simulink model "x12_agv"  (R2025a)
settings: Solver=VariableStepAuto  StartTime=0.0  StopTime=30  RelTol=1e-3
undefined symbols (not defined in the file): Ad, Bd, d_sel, K, kc_pos, kc_vel, p, ref_1, ref_10, ref_11, ref_12, ref_2, ref_3, ref_4, ref_5, ref_6, ref_7, ref_8, ref_9, Ts, x0, x0_1, x0_10, x0_11, x0_12, x0_2, x0_3, x0_4, x0_5, x0_6, x0_7, x0_8, x0_9
(part 1 of 2)
settings Model: Creator=pc  LastModifiedBy=pc

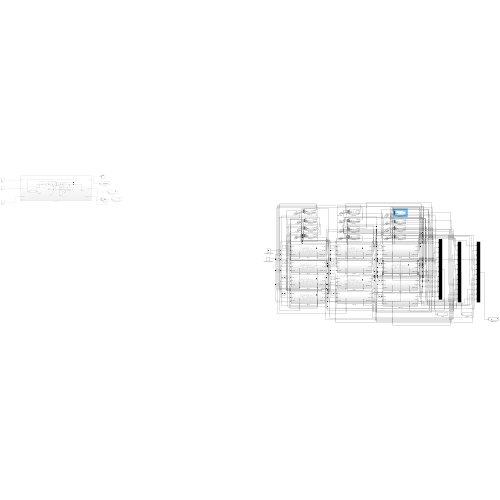
[thumbnail: Simulink's stored preview of the top-level diagram]
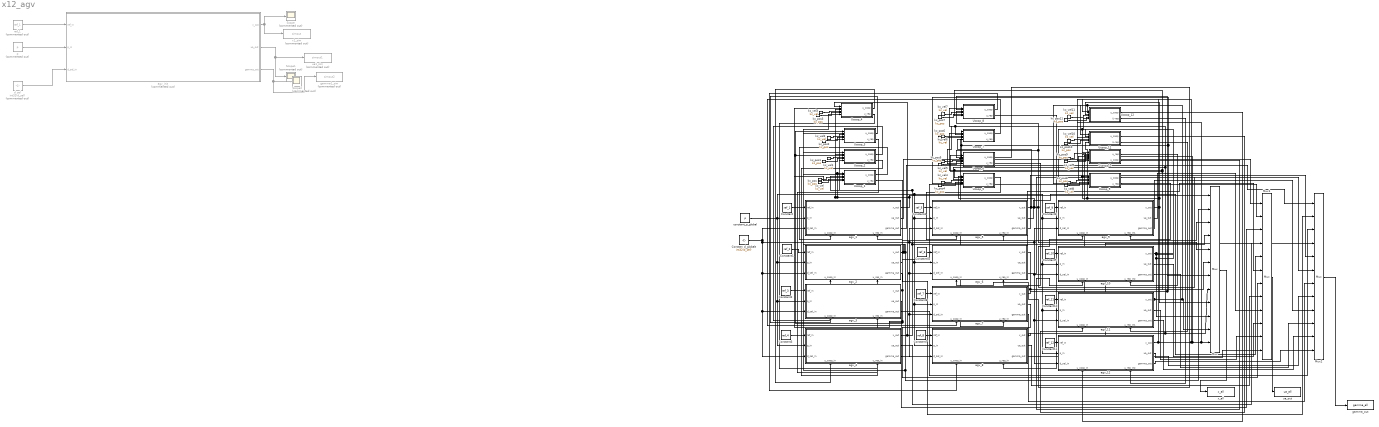
== system x12_agv ==
  Constan_d_globalt : Constant  Value=int32(d_sel)
  Constant : Constant  Value=ref_1
  Constant1 : Constant  Value=ref_2
  Constant10 : Constant  Value=ref_11
  Constant11 : Constant  Value=ref_12
  Constant2 : Constant  Value=ref_3
  Constant3 : Constant  Value=ref_4
  Constant4 : Constant  Value=ref_5
  Constant5 : Constant  Value=ref_6
  Constant6 : Constant  Value=ref_7
  Constant7 : Constant  Value=ref_8
  Constant8 : Constant  Value=ref_9
  Constant9 : Constant  Value=ref_10
  Mux : Mux  Inputs=12
  Mux1 : Mux  Inputs=12
  Mux2 : Mux  Inputs=12
  Scope : Scope  Commented=on
      settings: ActiveDisplayYMinimum=-8.609830640918906  ActiveDisplayYMaximum=10.643757487994291
  Scope1 : Scope  Commented=on
      settings: ActiveDisplayYMinimum=-1.4791031893143503  ActiveDisplayYMaximum=0.83872011794707424
  Scope2 : Scope  Commented=on
      settings: ActiveDisplayYMinimum=-0.20234469315895376  ActiveDisplayYMaximum=1.2446865568410463  DataLoggingVariableName=ScopeData2
  Ucoop_1 : Subsystem
  Ucoop_10 : Subsystem
  Ucoop_11 : Subsystem
  Ucoop_12 : Subsystem
  Ucoop_2 : Subsystem
  Ucoop_3 : Subsystem
  Ucoop_4 : Subsystem
  Ucoop_5 : Subsystem
  Ucoop_6 : Subsystem
  Ucoop_7 : Subsystem
  Ucoop_8 : Subsystem
  Ucoop_9 : Subsystem
  agv_1 : Subsystem
      settings: PortSchema="{\"entries\":[{\"content\":{\"sides\":[{\"content\":{\"connectorIds\":[\"In1\",\"In2\",\"In3\"]},\"type\":\"ConnectorPlacement.EquallySpacedRectSide\",\"uuid\":\"f08cf805-8739-441b-9df1-afc331da9c66\"},{\"content\":{\"connectorIds\":[\"Out1\",\"Out2\",\"Out3\"],\"side\":\"RIGHT\"},\"type\":\"ConnectorPlacement.EquallySpacedRectSide\",\"uuid\":\"8dfbec97-d8e8-49f2-8859-a95f098f15d4\"},{\"content\":{\"side\":\"TOP\"},\"type\":\"ConnectorPlacement.EquallySpacedRectSide\",\"uuid\":\"a9c3710a-c537-4e60-ba39-fa8e56fd912a\"},{\"content\":{\"connectorIds\":[\"In4\",\"In5\"],\"side\":\"BOTTOM\"},\"type\":\"ConnectorPlacement.EquallySpacedRectSide\",\"uuid\":\"8d7992a2-b8d6-4781-b503-987242c7d025\"}]},\"type\":\"ConnectorPlacement.EquallySpacedConnector\",\"uuid\":\"d7bc182e-c1cf-4fe9-ae71-f4bbcf9bd096\"}],\"packageUris\":[\"http://schema.mathworks.com/mf0/Connector/R2020b\"],\"version\":\"1.0\"}"
  agv_10 : Subsystem
      settings: PortSchema="{\"entries\":[{\"content\":{\"sides\":[{\"content\":{\"connectorIds\":[\"In1\",\"In2\",\"In3\"]},\"type\":\"ConnectorPlacement.EquallySpacedRectSide\",\"uuid\":\"f08cf805-8739-441b-9df1-afc331da9c66\"},{\"content\":{\"connectorIds\":[\"Out1\",\"Out2\",\"Out3\"],\"side\":\"RIGHT\"},\"type\":\"ConnectorPlacement.EquallySpacedRectSide\",\"uuid\":\"8dfbec97-d8e8-49f2-8859-a95f098f15d4\"},{\"content\":{\"side\":\"TOP\"},\"type\":\"ConnectorPlacement.EquallySpacedRectSide\",\"uuid\":\"a9c3710a-c537-4e60-ba39-fa8e56fd912a\"},{\"content\":{\"connectorIds\":[\"In4\",\"In5\"],\"side\":\"BOTTOM\"},\"type\":\"ConnectorPlacement.EquallySpacedRectSide\",\"uuid\":\"65549514-36e3-47a4-b89a-5d3e141dfba9\"}]},\"type\":\"ConnectorPlacement.EquallySpacedConnector\",\"uuid\":\"d7bc182e-c1cf-4fe9-ae71-f4bbcf9bd096\"}],\"packageUris\":[\"http://schema.mathworks.com/mf0/Connector/R2020b\"],\"version\":\"1.0\"}"
  agv_11 : Subsystem
      settings: PortSchema="{\"entries\":[{\"content\":{\"sides\":[{\"content\":{\"connectorIds\":[\"In1\",\"In2\",\"In3\"]},\"type\":\"ConnectorPlacement.EquallySpacedRectSide\",\"uuid\":\"f08cf805-8739-441b-9df1-afc331da9c66\"},{\"content\":{\"connectorIds\":[\"Out1\",\"Out2\",\"Out3\"],\"side\":\"RIGHT\"},\"type\":\"ConnectorPlacement.EquallySpacedRectSide\",\"uuid\":\"8dfbec97-d8e8-49f2-8859-a95f098f15d4\"},{\"content\":{\"side\":\"TOP\"},\"type\":\"ConnectorPlacement.EquallySpacedRectSide\",\"uuid\":\"a9c3710a-c537-4e60-ba39-fa8e56fd912a\"},{\"content\":{\"connectorIds\":[\"In4\",\"In5\"],\"side\":\"BOTTOM\"},\"type\":\"ConnectorPlacement.EquallySpacedRectSide\",\"uuid\":\"8d7992a2-b8d6-4781-b503-987242c7d025\"}]},\"type\":\"ConnectorPlacement.EquallySpacedConnector\",\"uuid\":\"d7bc182e-c1cf-4fe9-ae71-f4bbcf9bd096\"}],\"packageUris\":[\"http://schema.mathworks.com/mf0/Connector/R2020b\"],\"version\":\"1.0\"}"
  agv_12 : Subsystem
      settings: PortSchema="{\"entries\":[{\"content\":{\"sides\":[{\"content\":{\"connectorIds\":[\"In1\",\"In2\",\"In3\"]},\"type\":\"ConnectorPlacement.EquallySpacedRectSide\",\"uuid\":\"f08cf805-8739-441b-9df1-afc331da9c66\"},{\"content\":{\"connectorIds\":[\"Out1\",\"Out2\",\"Out3\"],\"side\":\"RIGHT\"},\"type\":\"ConnectorPlacement.EquallySpacedRectSide\",\"uuid\":\"8dfbec97-d8e8-49f2-8859-a95f098f15d4\"},{\"content\":{\"side\":\"TOP\"},\"type\":\"ConnectorPlacement.EquallySpacedRectSide\",\"uuid\":\"a9c3710a-c537-4e60-ba39-fa8e56fd912a\"},{\"content\":{\"connectorIds\":[\"In4\",\"In5\"],\"side\":\"BOTTOM\"},\"type\":\"ConnectorPlacement.EquallySpacedRectSide\",\"uuid\":\"8d7992a2-b8d6-4781-b503-987242c7d025\"}]},\"type\":\"ConnectorPlacement.EquallySpacedConnector\",\"uuid\":\"d7bc182e-c1cf-4fe9-ae71-f4bbcf9bd096\"}],\"packageUris\":[\"http://schema.mathworks.com/mf0/Connector/R2020b\"],\"version\":\"1.0\"}"
  agv_2 : Subsystem
      settings: PortSchema="{\"entries\":[{\"content\":{\"sides\":[{\"content\":{\"connectorIds\":[\"In1\",\"In2\",\"In3\"]},\"type\":\"ConnectorPlacement.EquallySpacedRectSide\",\"uuid\":\"f08cf805-8739-441b-9df1-afc331da9c66\"},{\"content\":{\"connectorIds\":[\"Out1\",\"Out2\",\"Out3\"],\"side\":\"RIGHT\"},\"type\":\"ConnectorPlacement.EquallySpacedRectSide\",\"uuid\":\"8dfbec97-d8e8-49f2-8859-a95f098f15d4\"},{\"content\":{\"side\":\"TOP\"},\"type\":\"ConnectorPlacement.EquallySpacedRectSide\",\"uuid\":\"a9c3710a-c537-4e60-ba39-fa8e56fd912a\"},{\"content\":{\"connectorIds\":[\"In4\",\"In5\"],\"side\":\"BOTTOM\"},\"type\":\"ConnectorPlacement.EquallySpacedRectSide\",\"uuid\":\"65549514-36e3-47a4-b89a-5d3e141dfba9\"}]},\"type\":\"ConnectorPlacement.EquallySpacedConnector\",\"uuid\":\"d7bc182e-c1cf-4fe9-ae71-f4bbcf9bd096\"}],\"packageUris\":[\"http://schema.mathworks.com/mf0/Connector/R2020b\"],\"version\":\"1.0\"}"
  agv_3 : Subsystem
      settings: PortSchema="{\"entries\":[{\"content\":{\"sides\":[{\"content\":{\"connectorIds\":[\"In1\",\"In2\",\"In3\"]},\"type\":\"ConnectorPlacement.EquallySpacedRectSide\",\"uuid\":\"f08cf805-8739-441b-9df1-afc331da9c66\"},{\"content\":{\"connectorIds\":[\"Out1\",\"Out2\",\"Out3\"],\"side\":\"RIGHT\"},\"type\":\"ConnectorPlacement.EquallySpacedRectSide\",\"uuid\":\"8dfbec97-d8e8-49f2-8859-a95f098f15d4\"},{\"content\":{\"side\":\"TOP\"},\"type\":\"ConnectorPlacement.EquallySpacedRectSide\",\"uuid\":\"a9c3710a-c537-4e60-ba39-fa8e56fd912a\"},{\"content\":{\"connectorIds\":[\"In4\",\"In5\"],\"side\":\"BOTTOM\"},\"type\":\"ConnectorPlacement.EquallySpacedRectSide\",\"uuid\":\"8d7992a2-b8d6-4781-b503-987242c7d025\"}]},\"type\":\"ConnectorPlacement.EquallySpacedConnector\",\"uuid\":\"d7bc182e-c1cf-4fe9-ae71-f4bbcf9bd096\"}],\"packageUris\":[\"http://schema.mathworks.com/mf0/Connector/R2020b\"],\"version\":\"1.0\"}"
  agv_4 : Subsystem
      settings: PortSchema="{\"entries\":[{\"content\":{\"sides\":[{\"content\":{\"connectorIds\":[\"In1\",\"In2\",\"In3\"]},\"type\":\"ConnectorPlacement.EquallySpacedRectSide\",\"uuid\":\"f08cf805-8739-441b-9df1-afc331da9c66\"},{\"content\":{\"connectorIds\":[\"Out1\",\"Out2\",\"Out3\"],\"side\":\"RIGHT\"},\"type\":\"ConnectorPlacement.EquallySpacedRectSide\",\"uuid\":\"8dfbec97-d8e8-49f2-8859-a95f098f15d4\"},{\"content\":{\"side\":\"TOP\"},\"type\":\"ConnectorPlacement.EquallySpacedRectSide\",\"uuid\":\"a9c3710a-c537-4e60-ba39-fa8e56fd912a\"},{\"content\":{\"connectorIds\":[\"In4\",\"In5\"],\"side\":\"BOTTOM\"},\"type\":\"ConnectorPlacement.EquallySpacedRectSide\",\"uuid\":\"8d7992a2-b8d6-4781-b503-987242c7d025\"}]},\"type\":\"ConnectorPlacement.EquallySpacedConnector\",\"uuid\":\"d7bc182e-c1cf-4fe9-ae71-f4bbcf9bd096\"}],\"packageUris\":[\"http://schema.mathworks.com/mf0/Connector/R2020b\"],\"version\":\"1.0\"}"
  agv_5 : Subsystem
      settings: PortSchema="{\"entries\":[{\"content\":{\"sides\":[{\"content\":{\"connectorIds\":[\"In1\",\"In2\",\"In3\"]},\"type\":\"ConnectorPlacement.EquallySpacedRectSide\",\"uuid\":\"f08cf805-8739-441b-9df1-afc331da9c66\"},{\"content\":{\"connectorIds\":[\"Out1\",\"Out2\",\"Out3\"],\"side\":\"RIGHT\"},\"type\":\"ConnectorPlacement.EquallySpacedRectSide\",\"uuid\":\"8dfbec97-d8e8-49f2-8859-a95f098f15d4\"},{\"content\":{\"side\":\"TOP\"},\"type\":\"ConnectorPlacement.EquallySpacedRectSide\",\"uuid\":\"a9c3710a-c537-4e60-ba39-fa8e56fd912a\"},{\"content\":{\"connectorIds\":[\"In4\",\"In5\"],\"side\":\"BOTTOM\"},\"type\":\"ConnectorPlacement.EquallySpacedRectSide\",\"uuid\":\"8d7992a2-b8d6-4781-b503-987242c7d025\"}]},\"type\":\"ConnectorPlacement.EquallySpacedConnector\",\"uuid\":\"d7bc182e-c1cf-4fe9-ae71-f4bbcf9bd096\"}],\"packageUris\":[\"http://schema.mathworks.com/mf0/Connector/R2020b\"],\"version\":\"1.0\"}"
  agv_6 : Subsystem
      settings: PortSchema="{\"entries\":[{\"content\":{\"sides\":[{\"content\":{\"connectorIds\":[\"In1\",\"In2\",\"In3\"]},\"type\":\"ConnectorPlacement.EquallySpacedRectSide\",\"uuid\":\"f08cf805-8739-441b-9df1-afc331da9c66\"},{\"content\":{\"connectorIds\":[\"Out1\",\"Out2\",\"Out3\"],\"side\":\"RIGHT\"},\"type\":\"ConnectorPlacement.EquallySpacedRectSide\",\"uuid\":\"8dfbec97-d8e8-49f2-8859-a95f098f15d4\"},{\"content\":{\"side\":\"TOP\"},\"type\":\"ConnectorPlacement.EquallySpacedRectSide\",\"uuid\":\"a9c3710a-c537-4e60-ba39-fa8e56fd912a\"},{\"content\":{\"connectorIds\":[\"In4\",\"In5\"],\"side\":\"BOTTOM\"},\"type\":\"ConnectorPlacement.EquallySpacedRectSide\",\"uuid\":\"65549514-36e3-47a4-b89a-5d3e141dfba9\"}]},\"type\":\"ConnectorPlacement.EquallySpacedConnector\",\"uuid\":\"d7bc182e-c1cf-4fe9-ae71-f4bbcf9bd096\"}],\"packageUris\":[\"http://schema.mathworks.com/mf0/Connector/R2020b\"],\"version\":\"1.0\"}"
  agv_7 : Subsystem
      settings: PortSchema="{\"entries\":[{\"content\":{\"sides\":[{\"content\":{\"connectorIds\":[\"In1\",\"In2\",\"In3\"]},\"type\":\"ConnectorPlacement.EquallySpacedRectSide\",\"uuid\":\"f08cf805-8739-441b-9df1-afc331da9c66\"},{\"content\":{\"connectorIds\":[\"Out1\",\"Out2\",\"Out3\"],\"side\":\"RIGHT\"},\"type\":\"ConnectorPlacement.EquallySpacedRectSide\",\"uuid\":\"8dfbec97-d8e8-49f2-8859-a95f098f15d4\"},{\"content\":{\"side\":\"TOP\"},\"type\":\"ConnectorPlacement.EquallySpacedRectSide\",\"uuid\":\"a9c3710a-c537-4e60-ba39-fa8e56fd912a\"},{\"content\":{\"connectorIds\":[\"In4\",\"In5\"],\"side\":\"BOTTOM\"},\"type\":\"ConnectorPlacement.EquallySpacedRectSide\",\"uuid\":\"8d7992a2-b8d6-4781-b503-987242c7d025\"}]},\"type\":\"ConnectorPlacement.EquallySpacedConnector\",\"uuid\":\"d7bc182e-c1cf-4fe9-ae71-f4bbcf9bd096\"}],\"packageUris\":[\"http://schema.mathworks.com/mf0/Connector/R2020b\"],\"version\":\"1.0\"}"
  agv_8 : Subsystem
      settings: PortSchema="{\"entries\":[{\"content\":{\"sides\":[{\"content\":{\"connectorIds\":[\"In1\",\"In2\",\"In3\"]},\"type\":\"ConnectorPlacement.EquallySpacedRectSide\",\"uuid\":\"f08cf805-8739-441b-9df1-afc331da9c66\"},{\"content\":{\"connectorIds\":[\"Out1\",\"Out2\",\"Out3\"],\"side\":\"RIGHT\"},\"type\":\"ConnectorPlacement.EquallySpacedRectSide\",\"uuid\":\"8dfbec97-d8e8-49f2-8859-a95f098f15d4\"},{\"content\":{\"side\":\"TOP\"},\"type\":\"ConnectorPlacement.EquallySpacedRectSide\",\"uuid\":\"a9c3710a-c537-4e60-ba39-fa8e56fd912a\"},{\"content\":{\"connectorIds\":[\"In4\",\"In5\"],\"side\":\"BOTTOM\"},\"type\":\"ConnectorPlacement.EquallySpacedRectSide\",\"uuid\":\"8d7992a2-b8d6-4781-b503-987242c7d025\"}]},\"type\":\"ConnectorPlacement.EquallySpacedConnector\",\"uuid\":\"d7bc182e-c1cf-4fe9-ae71-f4bbcf9bd096\"}],\"packageUris\":[\"http://schema.mathworks.com/mf0/Connector/R2020b\"],\"version\":\"1.0\"}"
  agv_9 : Subsystem
      settings: PortSchema="{\"entries\":[{\"content\":{\"sides\":[{\"content\":{\"connectorIds\":[\"In1\",\"In2\",\"In3\"]},\"type\":\"ConnectorPlacement.EquallySpacedRectSide\",\"uuid\":\"f08cf805-8739-441b-9df1-afc331da9c66\"},{\"content\":{\"connectorIds\":[\"Out1\",\"Out2\",\"Out3\"],\"side\":\"RIGHT\"},\"type\":\"ConnectorPlacement.EquallySpacedRectSide\",\"uuid\":\"8dfbec97-d8e8-49f2-8859-a95f098f15d4\"},{\"content\":{\"side\":\"TOP\"},\"type\":\"ConnectorPlacement.EquallySpacedRectSide\",\"uuid\":\"a9c3710a-c537-4e60-ba39-fa8e56fd912a\"},{\"content\":{\"connectorIds\":[\"In4\",\"In5\"],\"side\":\"BOTTOM\"},\"type\":\"ConnectorPlacement.EquallySpacedRectSide\",\"uuid\":\"8d7992a2-b8d6-4781-b503-987242c7d025\"}]},\"type\":\"ConnectorPlacement.EquallySpacedConnector\",\"uuid\":\"d7bc182e-c1cf-4fe9-ae71-f4bbcf9bd096\"}],\"packageUris\":[\"http://schema.mathworks.com/mf0/Connector/R2020b\"],\"version\":\"1.0\"}"
  agv_init : Subsystem  Commented=on
  constant_p_global : Constant  Value=p
  d_sel : Constant  Commented=on  Value=int32(d_sel)
  gamma1_sim : ToWorkspace  Commented=on  VariableName=simout2  SaveFormat=Timeseries  SampleTime=-1
  gamma_out : ToWorkspace  VariableName=gamma_all  SaveFormat=Timeseries  SampleTime=-1
  kc_pos{,1..11} (12 alike) : Constant  Value=kc_pos
  kc_vel{,1..11} (12 alike) : Constant  Value=kc_vel
  p : Constant  Commented=on  Value=p
  ref_1 : Constant  Commented=on  Value=ref_1
  ua1_sim : ToWorkspace  Commented=on  VariableName=simout1  SaveFormat=Timeseries  SampleTime=-1
  ua_out : ToWorkspace  VariableName=ua_all  SaveFormat=Timeseries  SampleTime=-1
  x1_sim : ToWorkspace  Commented=on  VariableName=simout  SaveFormat=Timeseries  SampleTime=-1
  x_all : ToWorkspace  VariableName=x_all  SaveFormat=Timeseries  SampleTime=-1
  wires:
  agv_init/1(x_out) -> Scope/1, x1_sim/1
  agv_init/2(ua_out) -> Scope1/1, ua1_sim/1
  agv_init/3(gamma_out) -> gamma1_sim/1, Scope2/1
  ref_1/1 -> agv_init/1(ref_in)
  p/1 -> agv_init/2(p_in)
  d_sel/1 -> agv_init/3(d_sel_in)
  constant_p_global/1 -> agv_9/2(p_in), agv_10/2(p_in), agv_12/2(p_in), agv_11/2(p_in), agv_5/2(p_in), agv_6/2(p_in), agv_8/2(p_in), agv_7/2(p_in), agv_1/2(p_in), agv_2/2(p_in), agv_4/2(p_in), agv_3/2(p_in)
  Constan_d_globalt/1 -> agv_5/3(d_sel_in), agv_9/3(d_sel_in), agv_10/3(d_sel_in), agv_12/3(d_sel_in), agv_11/3(d_sel_in), agv_6/3(d_sel_in), agv_8/3(d_sel_in), agv_7/3(d_sel_in), agv_2/3(d_sel_in), agv_4/3(d_sel_in), agv_3/3(d_sel_in), agv_1/3(d_sel_in)
  Constant/1 -> agv_1/1(ref_in)
  Constant1/1 -> agv_2/1(ref_in)
  Constant2/1 -> agv_3/1(ref_in)
  Constant3/1 -> agv_4/1(ref_in)
  Constant4/1 -> agv_5/1(ref_in)
  Constant5/1 -> agv_6/1(ref_in)
  Constant6/1 -> agv_7/1(ref_in)
  Constant7/1 -> agv_8/1(ref_in)
  Constant8/1 -> agv_9/1(ref_in)
  Constant9/1 -> agv_10/1(ref_in)
  Constant10/1 -> agv_11/1(ref_in)
  Constant11/1 -> agv_12/1(ref_in)
  agv_1/1(x_out) -> Ucoop_3/6(xj3), Ucoop_4/3(xj2), Ucoop_2/2(xj1), Ucoop_1/1(xi), Mux/1
  agv_2/1(x_out) -> Ucoop_4/6(xj3), Mux/2, Ucoop_3/2(xj1), Ucoop_1/2(xj1), Ucoop_2/1(xi)
  agv_3/1(x_out) -> Ucoop_1/6(xj3), Ucoop_4/2(xj1), Ucoop_3/1(xi), Ucoop_2/3(xj2), Mux/3
  agv_4/1(x_out) -> Ucoop_2/6(xj3), Ucoop_3/3(xj2), Mux/4, Ucoop_4/1(xi), Ucoop_1/3(xj2)
  agv_5/1(x_out) -> Ucoop_7/6(xj3), Ucoop_8/3(xj2), Ucoop_6/2(xj1), Mux/5, Ucoop_5/1(xi)
  agv_6/1(x_out) -> Ucoop_8/6(xj3), Ucoop_5/2(xj1), Ucoop_7/2(xj1), Ucoop_6/1(xi), Mux/6
  agv_7/1(x_out) -> Ucoop_5/6(xj3), Ucoop_7/1(xi), Ucoop_6/3(xj2), Ucoop_8/2(xj1), Mux/7
  agv_8/1(x_out) -> Ucoop_8/1(xi), Ucoop_5/3(xj2), Mux/8, Ucoop_6/6(xj3), Ucoop_7/3(xj2)
  agv_9/1(x_out) -> Ucoop_11/6(xj3), Ucoop_10/2(xj1), Ucoop_9/1(xi), Ucoop_12/3(xj2), Mux/9
  agv_10/1(x_out) -> Ucoop_12/6(xj3), Ucoop_11/2(xj1), Mux/10, Ucoop_10/1(xi), Ucoop_9/2(xj1)
  agv_11/1(x_out) -> Ucoop_9/6(xj3), Mux/11, Ucoop_12/2(xj1), Ucoop_11/1(xi), Ucoop_10/3(xj2)
  agv_12/1(x_out) -> Ucoop_10/6(xj3), Ucoop_12/1(xi), Ucoop_9/3(xj2), Ucoop_11/3(xj2), Mux/12
  Mux/1 -> x_all/1
  agv_1/2(ua_out) -> Mux1/1
  agv_2/2(ua_out) -> Mux1/2
  agv_3/2(ua_out) -> Mux1/3
  agv_4/2(ua_out) -> Mux1/4
  agv_5/2(ua_out) -> Mux1/5
  agv_6/2(ua_out) -> Mux1/6
  agv_7/2(ua_out) -> Mux1/7
  agv_8/2(ua_out) -> Mux1/8
  agv_9/2(ua_out) -> Mux1/9
  agv_10/2(ua_out) -> Mux1/10
  agv_11/2(ua_out) -> Mux1/11
  agv_12/2(ua_out) -> Mux1/12
  Mux1/1 -> ua_out/1
  agv_1/3(gamma_out) -> Mux2/1
  agv_2/3(gamma_out) -> Mux2/2
  agv_3/3(gamma_out) -> Mux2/3
  agv_4/3(gamma_out) -> Mux2/4
  agv_5/3(gamma_out) -> Mux2/5
  agv_6/3(gamma_out) -> Mux2/6
  agv_7/3(gamma_out) -> Mux2/7
  agv_8/3(gamma_out) -> Mux2/8
  agv_9/3(gamma_out) -> Mux2/9
  agv_10/3(gamma_out) -> Mux2/10
  agv_11/3(gamma_out) -> Mux2/11
  agv_12/3(gamma_out) -> Mux2/12
  Mux2/1 -> gamma_out/1
  Ucoop_1/1(u_coop) -> agv_1/4(u_coop_in)
  kc_pos/1 -> Ucoop_1/5(kc_pos)
  kc_vel/1 -> Ucoop_1/4(kc_vel)
  kc_pos1/1 -> Ucoop_2/5(kc_pos)
  kc_vel1/1 -> Ucoop_2/4(kc_vel)
  kc_vel2/1 -> Ucoop_3/4(kc_vel)
  kc_pos2/1 -> Ucoop_3/5(kc_pos)
  Ucoop_2/1(u_coop) -> agv_2/4(u_coop_in)
  Ucoop_3/1(u_coop) -> agv_3/4(u_coop_in)
  kc_vel3/1 -> Ucoop_4/4(kc_vel)
  kc_pos3/1 -> Ucoop_4/5(kc_pos)
  Ucoop_4/1(u_coop) -> agv_4/4(u_coop_in)
  kc_vel4/1 -> Ucoop_5/4(kc_vel)
  kc_pos4/1 -> Ucoop_5/5(kc_pos)
  kc_vel5/1 -> Ucoop_6/4(kc_vel)
  kc_pos5/1 -> Ucoop_6/5(kc_pos)
  kc_vel6/1 -> Ucoop_7/4(kc_vel)
  kc_pos6/1 -> Ucoop_7/5(kc_pos)
  kc_vel7/1 -> Ucoop_8/4(kc_vel)
  kc_pos7/1 -> Ucoop_8/5(kc_pos)
  kc_vel8/1 -> Ucoop_9/4(kc_vel)
  kc_pos8/1 -> Ucoop_9/5(kc_pos)
  kc_vel9/1 -> Ucoop_10/4(kc_vel)
  kc_pos9/1 -> Ucoop_10/5(kc_pos)
  kc_vel10/1 -> Ucoop_11/4(kc_vel)
  kc_pos10/1 -> Ucoop_11/5(kc_pos)
  kc_vel11/1 -> Ucoop_12/4(kc_vel)
  kc_pos11/1 -> Ucoop_12/5(kc_pos)
  Ucoop_5/1(u_coop) -> agv_5/4(u_coop_in)
  Ucoop_6/1(u_coop) -> agv_6/4(u_coop_in)
  Ucoop_7/1(u_coop) -> agv_7/4(u_coop_in)
  Ucoop_8/1(u_coop) -> agv_8/4(u_coop_in)
  Ucoop_9/1(u_coop) -> agv_9/4(u_coop_in)
  Ucoop_10/2(u_coop) -> agv_10/4(u_coop_in)
  Ucoop_11/1(u_coop) -> agv_11/4(u_coop_in)
  Ucoop_12/1(u_coop) -> agv_12/4(u_coop_in)
  Ucoop_1/2(u_rep) -> agv_1/5(u_rep_in)
  Ucoop_2/2(u_rep) -> agv_2/5(u_rep_in)
  Ucoop_3/2(u_rep) -> agv_3/5(u_rep_in)
  Ucoop_4/2(u_rep) -> agv_4/5(u_rep_in)
  Ucoop_5/2(u_rep) -> agv_5/5(u_rep_in)
  Ucoop_6/2(u_rep) -> agv_6/5(u_rep_in)
  Ucoop_7/2(u_rep) -> agv_7/5(u_rep_in)
  Ucoop_8/2(u_rep) -> agv_8/5(u_rep_in)
  Ucoop_9/2(u_rep) -> agv_9/5(u_rep_in1)
  Ucoop_10/1(u_rep) -> agv_10/5(u_rep_in2)
  Ucoop_11/2(U-rep) -> agv_11/5(u_rep_in1)
  Ucoop_12/2(U-rep) -> agv_12/5(u_rep_in2)

== system x12_agv/Ucoop_1 ==
  xi : Inport
  xj1 : Inport  Port=2
  xj2 : Inport  Port=3
  kc_vel : Inport  Port=4
  kc_pos : Inport  Port=5
  xj3 : Inport  Port=6
  MATLAB Function : MATLAB Function  TreatAsAtomicUnit=on
  u_coop : Outport
  u_rep : Outport  Port=2
  wires:
  MATLAB Function/1(u_coop) -> u_coop/1
  xi/1 -> MATLAB Function/1(xi)
  xj1/1 -> MATLAB Function/2(xj1)
  xj2/1 -> MATLAB Function/3(xj2)
  kc_pos/1 -> MATLAB Function/5(kc_pos)
  kc_vel/1 -> MATLAB Function/6(kc_vel)
  MATLAB Function/2(u_rep) -> u_rep/1
  xj3/1 -> MATLAB Function/4(xj3)

== system x12_agv/Ucoop_10 ==
  xi : Inport
  xj1 : Inport  Port=2
  xj2 : Inport  Port=3
  kc_vel : Inport  Port=4
  kc_pos : Inport  Port=5
  xj3 : Inport  Port=6
  MATLAB Function : MATLAB Function  TreatAsAtomicUnit=on
  u_rep : Outport
  u_coop : Outport  Port=2
  wires:
  MATLAB Function/1(u_coop) -> u_coop/1
  xi/1 -> MATLAB Function/1(xi)
  xj1/1 -> MATLAB Function/2(xj1)
  xj2/1 -> MATLAB Function/3(xj2)
  kc_pos/1 -> MATLAB Function/5(kc_pos)
  kc_vel/1 -> MATLAB Function/6(kc_vel)
  MATLAB Function/2(u_rep) -> u_rep/1
  xj3/1 -> MATLAB Function/4(xj3)

== system x12_agv/Ucoop_11 ==
  xi : Inport
  xj1 : Inport  Port=2
  xj2 : Inport  Port=3
  kc_vel : Inport  Port=4
  kc_pos : Inport  Port=5
  xj3 : Inport  Port=6
  MATLAB Function : MATLAB Function  TreatAsAtomicUnit=on
  u_coop : Outport
  U-rep : Outport  Port=2
  wires:
  MATLAB Function/1(u_coop) -> u_coop/1
  xi/1 -> MATLAB Function/1(xi)
  xj1/1 -> MATLAB Function/2(xj1)
  xj2/1 -> MATLAB Function/3(xj2)
  kc_pos/1 -> MATLAB Function/5(kc_pos)
  kc_vel/1 -> MATLAB Function/6(kc_vel)
  MATLAB Function/2(u_rep) -> U-rep/1
  xj3/1 -> MATLAB Function/4(xj3)

== system x12_agv/Ucoop_12 ==
  xi : Inport
  xj1 : Inport  Port=2
  xj2 : Inport  Port=3
  kc_vel : Inport  Port=4
  kc_pos : Inport  Port=5
  xj3 : Inport  Port=6
  MATLAB Function : MATLAB Function  TreatAsAtomicUnit=on
  u_coop : Outport
  U-rep : Outport  Port=2
  wires:
  MATLAB Function/1(u_coop) -> u_coop/1
  xi/1 -> MATLAB Function/1(xi)
  xj1/1 -> MATLAB Function/2(xj1)
  xj2/1 -> MATLAB Function/3(xj2)
  kc_pos/1 -> MATLAB Function/5(kc_pos)
  kc_vel/1 -> MATLAB Function/6(kc_vel)
  MATLAB Function/2(u_rep) -> U-rep/1
  xj3/1 -> MATLAB Function/4(xj3)

== system x12_agv/Ucoop_2 ==
  xi : Inport
  xj1 : Inport  Port=2
  xj2 : Inport  Port=3
  kc_vel : Inport  Port=4
  kc_pos : Inport  Port=5
  xj3 : Inport  Port=6
  MATLAB Function : MATLAB Function  TreatAsAtomicUnit=on
  u_coop : Outport
  u_rep : Outport  Port=2
  wires:
  MATLAB Function/1(u_coop) -> u_coop/1
  xi/1 -> MATLAB Function/1(xi)
  xj1/1 -> MATLAB Function/2(xj1)
  xj2/1 -> MATLAB Function/3(xj2)
  kc_pos/1 -> MATLAB Function/5(kc_pos)
  kc_vel/1 -> MATLAB Function/6(kc_vel)
  MATLAB Function/2(u_rep) -> u_rep/1
  xj3/1 -> MATLAB Function/4(xj3)

== system x12_agv/Ucoop_3 ==
  xi : Inport
  xj1 : Inport  Port=2
  xj2 : Inport  Port=3
  kc_vel : Inport  Port=4
  kc_pos : Inport  Port=5
  xj3 : Inport  Port=6
  MATLAB Function : MATLAB Function  TreatAsAtomicUnit=on
  u_coop : Outport
  u_rep : Outport  Port=2
  wires:
  MATLAB Function/1(u_coop) -> u_coop/1
  xi/1 -> MATLAB Function/1(xi)
  xj1/1 -> MATLAB Function/2(xj1)
  xj2/1 -> MATLAB Function/3(xj2)
  kc_pos/1 -> MATLAB Function/5(kc_pos)
  kc_vel/1 -> MATLAB Function/6(kc_vel)
  MATLAB Function/2(u_rep) -> u_rep/1
  xj3/1 -> MATLAB Function/4(xj3)

== system x12_agv/Ucoop_4 ==
  xi : Inport
  xj1 : Inport  Port=2
  xj2 : Inport  Port=3
  kc_vel : Inport  Port=4
  kc_pos : Inport  Port=5
  xj3 : Inport  Port=6
  MATLAB Function : MATLAB Function  TreatAsAtomicUnit=on
  u_coop : Outport
  u_rep : Outport  Port=2
  wires:
  MATLAB Function/1(u_coop) -> u_coop/1
  xi/1 -> MATLAB Function/1(xi)
  xj1/1 -> MATLAB Function/2(xj1)
  xj2/1 -> MATLAB Function/3(xj2)
  kc_pos/1 -> MATLAB Function/5(kc_pos)
  kc_vel/1 -> MATLAB Function/6(kc_vel)
  MATLAB Function/2(u_rep) -> u_rep/1
  xj3/1 -> MATLAB Function/4(xj3)

== system x12_agv/Ucoop_5 ==
  xi : Inport
  xj1 : Inport  Port=2
  xj2 : Inport  Port=3
  kc_vel : Inport  Port=4
  kc_pos : Inport  Port=5
  xj3 : Inport  Port=6
  MATLAB Function : MATLAB Function  TreatAsAtomicUnit=on
  u_coop : Outport
  u_rep : Outport  Port=2
  wires:
  MATLAB Function/1(u_coop) -> u_coop/1
  xi/1 -> MATLAB Function/1(xi)
  xj1/1 -> MATLAB Function/2(xj1)
  xj2/1 -> MATLAB Function/3(xj2)
  kc_pos/1 -> MATLAB Function/5(kc_pos)
  kc_vel/1 -> MATLAB Function/6(kc_vel)
  MATLAB Function/2(u_rep) -> u_rep/1
  xj3/1 -> MATLAB Function/4(xj3)

== system x12_agv/Ucoop_6 ==
  xi : Inport
  xj1 : Inport  Port=2
  xj2 : Inport  Port=3
  kc_vel : Inport  Port=4
  kc_pos : Inport  Port=5
  xj3 : Inport  Port=6
  MATLAB Function : MATLAB Function  TreatAsAtomicUnit=on
  u_coop : Outport
  u_rep : Outport  Port=2
  wires:
  MATLAB Function/1(u_coop) -> u_coop/1
  xi/1 -> MATLAB Function/1(xi)
  xj1/1 -> MATLAB Function/2(xj1)
  xj2/1 -> MATLAB Function/3(xj2)
  kc_pos/1 -> MATLAB Function/5(kc_pos)
  kc_vel/1 -> MATLAB Function/6(kc_vel)
  MATLAB Function/2(u_rep) -> u_rep/1
  xj3/1 -> MATLAB Function/4(xj3)

== system x12_agv/Ucoop_7 ==
  xi : Inport
  xj1 : Inport  Port=2
  xj2 : Inport  Port=3
  kc_vel : Inport  Port=4
  kc_pos : Inport  Port=5
  xj3 : Inport  Port=6
  MATLAB Function : MATLAB Function  TreatAsAtomicUnit=on
  u_coop : Outport
  u_rep : Outport  Port=2
  wires:
  MATLAB Function/1(u_coop) -> u_coop/1
  xi/1 -> MATLAB Function/1(xi)
  xj1/1 -> MATLAB Function/2(xj1)
  xj2/1 -> MATLAB Function/3(xj2)
  kc_pos/1 -> MATLAB Function/5(kc_pos)
  kc_vel/1 -> MATLAB Function/6(kc_vel)
  MATLAB Function/2(u_rep) -> u_rep/1
  xj3/1 -> MATLAB Function/4(xj3)

== system x12_agv/Ucoop_8 ==
  xi : Inport
  xj1 : Inport  Port=2
  xj2 : Inport  Port=3
  kc_vel : Inport  Port=4
  kc_pos : Inport  Port=5
  xj3 : Inport  Port=6
  MATLAB Function : MATLAB Function  TreatAsAtomicUnit=on
  u_coop : Outport
  u_rep : Outport  Port=2
  wires:
  MATLAB Function/1(u_coop) -> u_coop/1
  xi/1 -> MATLAB Function/1(xi)
  xj1/1 -> MATLAB Function/2(xj1)
  xj2/1 -> MATLAB Function/3(xj2)
  kc_pos/1 -> MATLAB Function/5(kc_pos)
  kc_vel/1 -> MATLAB Function/6(kc_vel)
  MATLAB Function/2(u_rep) -> u_rep/1
  xj3/1 -> MATLAB Function/4(xj3)

== system x12_agv/Ucoop_9 ==
  xi : Inport
  xj1 : Inport  Port=2
  xj2 : Inport  Port=3
  kc_vel : Inport  Port=4
  kc_pos : Inport  Port=5
  xj3 : Inport  Port=6
  MATLAB Function : MATLAB Function  TreatAsAtomicUnit=on
  u_coop : Outport
  u_rep : Outport  Port=2
  wires:
  MATLAB Function/1(u_coop) -> u_coop/1
  xi/1 -> MATLAB Function/1(xi)
  xj1/1 -> MATLAB Function/2(xj1)
  xj2/1 -> MATLAB Function/3(xj2)
  kc_pos/1 -> MATLAB Function/5(kc_pos)
  kc_vel/1 -> MATLAB Function/6(kc_vel)
  MATLAB Function/2(u_rep) -> u_rep/1
  xj3/1 -> MATLAB Function/4(xj3)

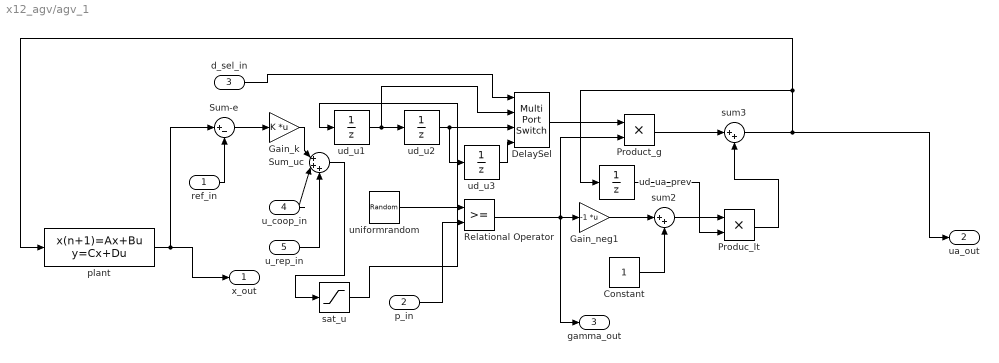
== system x12_agv/agv_1 ==
  ref_in : Inport
  p_in : Inport  Port=2
  d_sel_in : Inport  Port=3
  u_coop_in : Inport  Port=4
  u_rep_in : Inport  Port=5
  Constant : Constant
  DelaySel : MultiPortSwitch  DataPortOrder=Specify indices  DiagnosticForDefault=None  SaturateOnIntegerOverflow=off  InputSameDT=off
  Gain_k : Gain  Gain=K  Multiplication=Matrix(K*u)
  Gain_neg1 : Gain  Gain=-1  Multiplication=Matrix(K*u)
  Produc_lt : Product
  Product_g : Product
  Relational Operator : RelationalOperator  OutDataTypeStr=boolean  RndMeth=Simplest  InputSameDT=off
  Sum-e : Sum  Inputs=|+-
  Sum_uc : Sum  Inputs=|+++
  plant : DiscreteStateSpace  A=Ad  B=Bd  C=eye(4)  D=zeros(4,2)  InitialCondition=x0_1  SampleTime=Ts
  sat_u : Saturate  UpperLimit=1.0  LowerLimit=-1.0
  sum2 : Sum  Inputs=|++
  sum3 : Sum  Inputs=|++
  ud_u1 : UnitDelay  InitialCondition=[0;0]  SampleTime=Ts  HasFrameUpgradeWarning=on
  ud_u2 : UnitDelay  InitialCondition=[0;0]  SampleTime=Ts  HasFrameUpgradeWarning=on
  ud_u3 : UnitDelay  InitialCondition=[0;0]  SampleTime=Ts  HasFrameUpgradeWarning=on
  ud_ua_prev : UnitDelay  InitialCondition=[0;0]  SampleTime=Ts  HasFrameUpgradeWarning=on
  uniformrandom : UniformRandomNumber  Minimum=0  SampleTime=Ts
  x_out : Outport
  ua_out : Outport  Port=2
  gamma_out : Outport  Port=3
  wires:
  ud_u1/1 -> ud_u2/1, DelaySel/2
  Relational Operator/1 -> gamma_out/1, Product_g/2, Gain_neg1/1
  ud_u3/1 -> DelaySel/4
  plant/1 -> Sum-e/1, x_out/1
  Produc_lt/1 -> sum3/2
  sum2/1 -> Produc_lt/1
  ud_ua_prev/1 -> Produc_lt/2
  Constant/1 -> sum2/2
  Gain_neg1/1 -> sum2/1
  DelaySel/1 -> Product_g/1
  Product_g/1 -> sum3/1
  ud_u2/1 -> ud_u3/1, DelaySel/3
  Sum-e/1 -> Gain_k/1
  sum3/1 -> ud_ua_prev/1, plant/1, ua_out/1
  uniformrandom/1 -> Relational Operator/1
  ref_in/1 -> Sum-e/2
  p_in/1 -> Relational Operator/2
  d_sel_in/1 -> DelaySel/1
  Gain_k/1 -> Sum_uc/1
  u_coop_in/1 -> Sum_uc/2
  u_rep_in/1 -> Sum_uc/3
  Sum_uc/1 -> sat_u/1
  sat_u/1 -> ud_u1/1

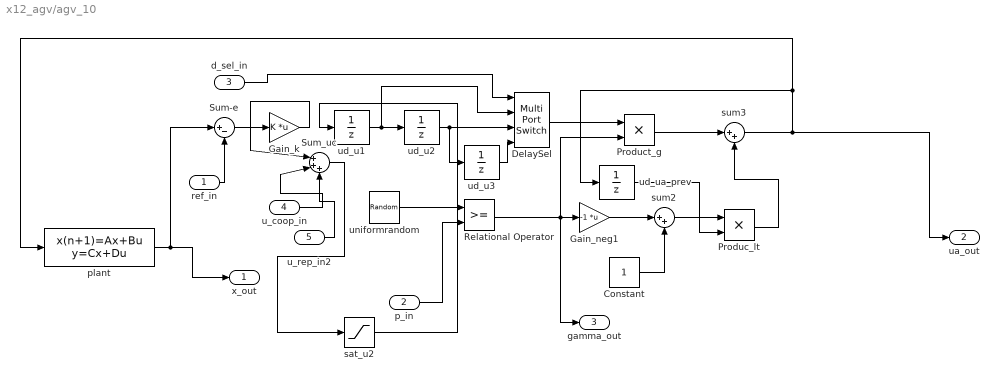
== system x12_agv/agv_10 ==
  ref_in : Inport
  p_in : Inport  Port=2
  d_sel_in : Inport  Port=3
  u_coop_in : Inport  Port=4
  u_rep_in2 : Inport  Port=5
  Constant : Constant
  DelaySel : MultiPortSwitch  DataPortOrder=Specify indices  DiagnosticForDefault=None  SaturateOnIntegerOverflow=off  InputSameDT=off
  Gain_k : Gain  Gain=K  Multiplication=Matrix(K*u)
  Gain_neg1 : Gain  Gain=-1  Multiplication=Matrix(K*u)
  Produc_lt : Product
  Product_g : Product
  Relational Operator : RelationalOperator  OutDataTypeStr=boolean  RndMeth=Simplest  InputSameDT=off
  Sum-e : Sum  Inputs=|+-
  Sum_uc : Sum  Inputs=|+++
  plant : DiscreteStateSpace  A=Ad  B=Bd  C=eye(4)  D=zeros(4,2)  InitialCondition=x0_10  SampleTime=Ts
  sat_u2 : Saturate  UpperLimit=1.0  LowerLimit=-1.0
  sum2 : Sum  Inputs=|++
  sum3 : Sum  Inputs=|++
  ud_u1 : UnitDelay  InitialCondition=[0;0]  SampleTime=Ts  HasFrameUpgradeWarning=on
  ud_u2 : UnitDelay  InitialCondition=[0;0]  SampleTime=Ts  HasFrameUpgradeWarning=on
  ud_u3 : UnitDelay  InitialCondition=[0;0]  SampleTime=Ts  HasFrameUpgradeWarning=on
  ud_ua_prev : UnitDelay  InitialCondition=[0;0]  SampleTime=Ts  HasFrameUpgradeWarning=on
  uniformrandom : UniformRandomNumber  Minimum=0  SampleTime=Ts
  x_out : Outport
  ua_out : Outport  Port=2
  gamma_out : Outport  Port=3
  wires:
  ud_u1/1 -> ud_u2/1, DelaySel/2
  Relational Operator/1 -> gamma_out/1, Product_g/2, Gain_neg1/1
  ud_u3/1 -> DelaySel/4
  plant/1 -> Sum-e/1, x_out/1
  Produc_lt/1 -> sum3/2
  sum2/1 -> Produc_lt/1
  ud_ua_prev/1 -> Produc_lt/2
  Constant/1 -> sum2/2
  Gain_neg1/1 -> sum2/1
  DelaySel/1 -> Product_g/1
  Product_g/1 -> sum3/1
  ud_u2/1 -> ud_u3/1, DelaySel/3
  Sum-e/1 -> Gain_k/1
  sum3/1 -> ud_ua_prev/1, plant/1, ua_out/1
  uniformrandom/1 -> Relational Operator/1
  ref_in/1 -> Sum-e/2
  p_in/1 -> Relational Operator/2
  d_sel_in/1 -> DelaySel/1
  Gain_k/1 -> Sum_uc/1
  u_coop_in/1 -> Sum_uc/2
  Sum_uc/1 -> sat_u2/1
  sat_u2/1 -> ud_u1/1
  u_rep_in2/1 -> Sum_uc/3

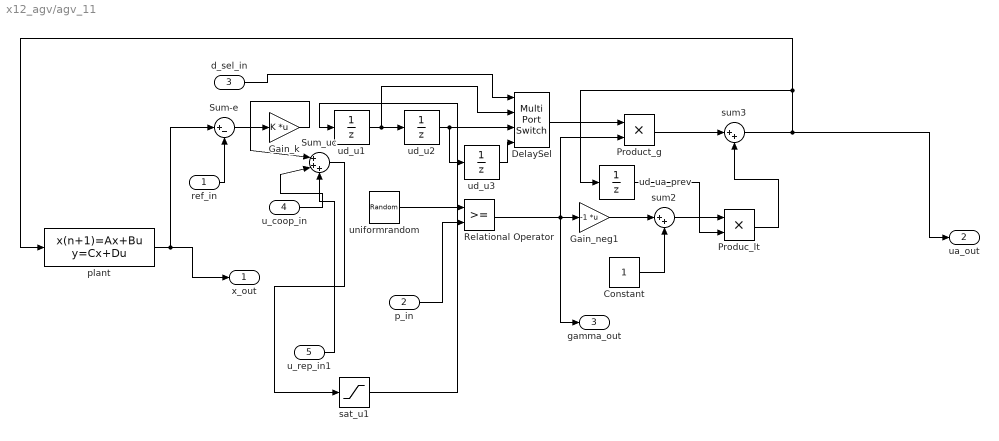
== system x12_agv/agv_11 ==
  ref_in : Inport
  p_in : Inport  Port=2
  d_sel_in : Inport  Port=3
  u_coop_in : Inport  Port=4
  u_rep_in1 : Inport  Port=5
  Constant : Constant
  DelaySel : MultiPortSwitch  DataPortOrder=Specify indices  DiagnosticForDefault=None  SaturateOnIntegerOverflow=off  InputSameDT=off
  Gain_k : Gain  Gain=K  Multiplication=Matrix(K*u)
  Gain_neg1 : Gain  Gain=-1  Multiplication=Matrix(K*u)
  Produc_lt : Product
  Product_g : Product
  Relational Operator : RelationalOperator  OutDataTypeStr=boolean  RndMeth=Simplest  InputSameDT=off
  Sum-e : Sum  Inputs=|+-
  Sum_uc : Sum  Inputs=|+++
  plant : DiscreteStateSpace  A=Ad  B=Bd  C=eye(4)  D=zeros(4,2)  InitialCondition=x0_11  SampleTime=Ts
  sat_u1 : Saturate  UpperLimit=1.0  LowerLimit=-1.0
  sum2 : Sum  Inputs=|++
  sum3 : Sum  Inputs=|++
  ud_u1 : UnitDelay  InitialCondition=[0;0]  SampleTime=Ts  HasFrameUpgradeWarning=on
  ud_u2 : UnitDelay  InitialCondition=[0;0]  SampleTime=Ts  HasFrameUpgradeWarning=on
  ud_u3 : UnitDelay  InitialCondition=[0;0]  SampleTime=Ts  HasFrameUpgradeWarning=on
  ud_ua_prev : UnitDelay  InitialCondition=[0;0]  SampleTime=Ts  HasFrameUpgradeWarning=on
  uniformrandom : UniformRandomNumber  Minimum=0  SampleTime=Ts
  x_out : Outport
  ua_out : Outport  Port=2
  gamma_out : Outport  Port=3
  wires:
  ud_u1/1 -> ud_u2/1, DelaySel/2
  Relational Operator/1 -> gamma_out/1, Product_g/2, Gain_neg1/1
  ud_u3/1 -> DelaySel/4
  plant/1 -> Sum-e/1, x_out/1
  Produc_lt/1 -> sum3/2
  sum2/1 -> Produc_lt/1
  ud_ua_prev/1 -> Produc_lt/2
  Constant/1 -> sum2/2
  Gain_neg1/1 -> sum2/1
  DelaySel/1 -> Product_g/1
  Product_g/1 -> sum3/1
  ud_u2/1 -> ud_u3/1, DelaySel/3
  Sum-e/1 -> Gain_k/1
  sum3/1 -> ud_ua_prev/1, plant/1, ua_out/1
  uniformrandom/1 -> Relational Operator/1
  ref_in/1 -> Sum-e/2
  p_in/1 -> Relational Operator/2
  d_sel_in/1 -> DelaySel/1
  Gain_k/1 -> Sum_uc/1
  u_coop_in/1 -> Sum_uc/2
  Sum_uc/1 -> sat_u1/1
  sat_u1/1 -> ud_u1/1
  u_rep_in1/1 -> Sum_uc/3

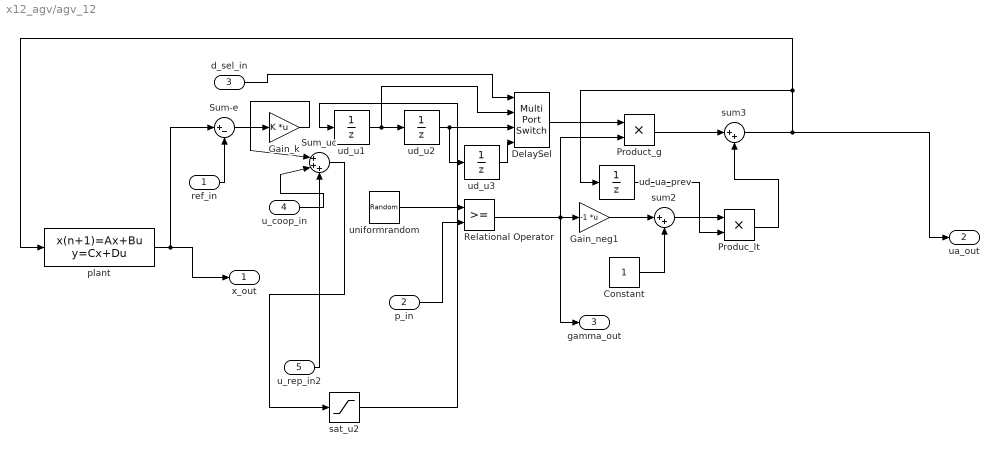
== system x12_agv/agv_12 ==
  ref_in : Inport
  p_in : Inport  Port=2
  d_sel_in : Inport  Port=3
  u_coop_in : Inport  Port=4
  u_rep_in2 : Inport  Port=5
  Constant : Constant
  DelaySel : MultiPortSwitch  DataPortOrder=Specify indices  DiagnosticForDefault=None  SaturateOnIntegerOverflow=off  InputSameDT=off
  Gain_k : Gain  Gain=K  Multiplication=Matrix(K*u)
  Gain_neg1 : Gain  Gain=-1  Multiplication=Matrix(K*u)
  Produc_lt : Product
  Product_g : Product
  Relational Operator : RelationalOperator  OutDataTypeStr=boolean  RndMeth=Simplest  InputSameDT=off
  Sum-e : Sum  Inputs=|+-
  Sum_uc : Sum  Inputs=|+++
  plant : DiscreteStateSpace  A=Ad  B=Bd  C=eye(4)  D=zeros(4,2)  InitialCondition=x0_12  SampleTime=Ts
  sat_u2 : Saturate  UpperLimit=1.0  LowerLimit=-1.0
  sum2 : Sum  Inputs=|++
  sum3 : Sum  Inputs=|++
  ud_u1 : UnitDelay  InitialCondition=[0;0]  SampleTime=Ts  HasFrameUpgradeWarning=on
  ud_u2 : UnitDelay  InitialCondition=[0;0]  SampleTime=Ts  HasFrameUpgradeWarning=on
  ud_u3 : UnitDelay  InitialCondition=[0;0]  SampleTime=Ts  HasFrameUpgradeWarning=on
  ud_ua_prev : UnitDelay  InitialCondition=[0;0]  SampleTime=Ts  HasFrameUpgradeWarning=on
  uniformrandom : UniformRandomNumber  Minimum=0  SampleTime=Ts
  x_out : Outport
  ua_out : Outport  Port=2
  gamma_out : Outport  Port=3
  wires:
  ud_u1/1 -> ud_u2/1, DelaySel/2
  Relational Operator/1 -> gamma_out/1, Product_g/2, Gain_neg1/1
  ud_u3/1 -> DelaySel/4
  plant/1 -> Sum-e/1, x_out/1
  Produc_lt/1 -> sum3/2
  sum2/1 -> Produc_lt/1
  ud_ua_prev/1 -> Produc_lt/2
  Constant/1 -> sum2/2
  Gain_neg1/1 -> sum2/1
  DelaySel/1 -> Product_g/1
  Product_g/1 -> sum3/1
  ud_u2/1 -> ud_u3/1, DelaySel/3
  Sum-e/1 -> Gain_k/1
  sum3/1 -> ud_ua_prev/1, plant/1, ua_out/1
  uniformrandom/1 -> Relational Operator/1
  ref_in/1 -> Sum-e/2
  p_in/1 -> Relational Operator/2
  d_sel_in/1 -> DelaySel/1
  Gain_k/1 -> Sum_uc/1
  u_coop_in/1 -> Sum_uc/2
  u_rep_in2/1 -> Sum_uc/3
  Sum_uc/1 -> sat_u2/1
  sat_u2/1 -> ud_u1/1

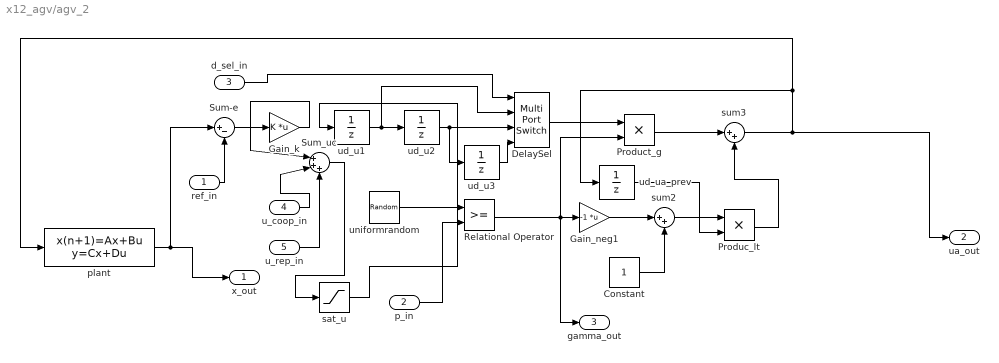
== system x12_agv/agv_2 ==
  ref_in : Inport
  p_in : Inport  Port=2
  d_sel_in : Inport  Port=3
  u_coop_in : Inport  Port=4
  u_rep_in : Inport  Port=5
  Constant : Constant
  DelaySel : MultiPortSwitch  DataPortOrder=Specify indices  DiagnosticForDefault=None  SaturateOnIntegerOverflow=off  InputSameDT=off
  Gain_k : Gain  Gain=K  Multiplication=Matrix(K*u)
  Gain_neg1 : Gain  Gain=-1  Multiplication=Matrix(K*u)
  Produc_lt : Product
  Product_g : Product
  Relational Operator : RelationalOperator  OutDataTypeStr=boolean  RndMeth=Simplest  InputSameDT=off
  Sum-e : Sum  Inputs=|+-
  Sum_uc : Sum  Inputs=|+++
  plant : DiscreteStateSpace  A=Ad  B=Bd  C=eye(4)  D=zeros(4,2)  InitialCondition=x0_2  SampleTime=Ts
  sat_u : Saturate  UpperLimit=1.0  LowerLimit=-1.0
  sum2 : Sum  Inputs=|++
  sum3 : Sum  Inputs=|++
  ud_u1 : UnitDelay  InitialCondition=[0;0]  SampleTime=Ts  HasFrameUpgradeWarning=on
  ud_u2 : UnitDelay  InitialCondition=[0;0]  SampleTime=Ts  HasFrameUpgradeWarning=on
  ud_u3 : UnitDelay  InitialCondition=[0;0]  SampleTime=Ts  HasFrameUpgradeWarning=on
  ud_ua_prev : UnitDelay  InitialCondition=[0;0]  SampleTime=Ts  HasFrameUpgradeWarning=on
  uniformrandom : UniformRandomNumber  Minimum=0  SampleTime=Ts
  x_out : Outport
  ua_out : Outport  Port=2
  gamma_out : Outport  Port=3
  wires:
  ud_u1/1 -> ud_u2/1, DelaySel/2
  Relational Operator/1 -> gamma_out/1, Product_g/2, Gain_neg1/1
  ud_u3/1 -> DelaySel/4
  plant/1 -> Sum-e/1, x_out/1
  Produc_lt/1 -> sum3/2
  sum2/1 -> Produc_lt/1
  ud_ua_prev/1 -> Produc_lt/2
  Constant/1 -> sum2/2
  Gain_neg1/1 -> sum2/1
  DelaySel/1 -> Product_g/1
  Product_g/1 -> sum3/1
  ud_u2/1 -> ud_u3/1, DelaySel/3
  Sum-e/1 -> Gain_k/1
  sum3/1 -> ud_ua_prev/1, plant/1, ua_out/1
  uniformrandom/1 -> Relational Operator/1
  ref_in/1 -> Sum-e/2
  p_in/1 -> Relational Operator/2
  d_sel_in/1 -> DelaySel/1
  Gain_k/1 -> Sum_uc/1
  u_coop_in/1 -> Sum_uc/2
  sat_u/1 -> ud_u1/1
  Sum_uc/1 -> sat_u/1
  u_rep_in/1 -> Sum_uc/3

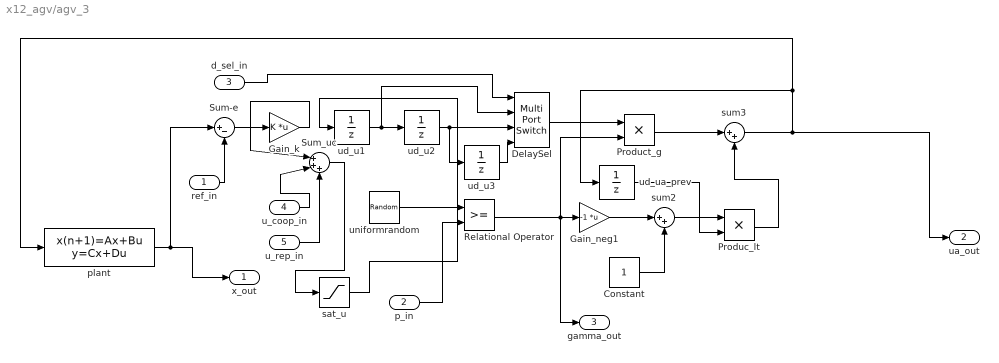
== system x12_agv/agv_3 ==
  ref_in : Inport
  p_in : Inport  Port=2
  d_sel_in : Inport  Port=3
  u_coop_in : Inport  Port=4
  u_rep_in : Inport  Port=5
  Constant : Constant
  DelaySel : MultiPortSwitch  DataPortOrder=Specify indices  DiagnosticForDefault=None  SaturateOnIntegerOverflow=off  InputSameDT=off
  Gain_k : Gain  Gain=K  Multiplication=Matrix(K*u)
  Gain_neg1 : Gain  Gain=-1  Multiplication=Matrix(K*u)
  Produc_lt : Product
  Product_g : Product
  Relational Operator : RelationalOperator  OutDataTypeStr=boolean  RndMeth=Simplest  InputSameDT=off
  Sum-e : Sum  Inputs=|+-
  Sum_uc : Sum  Inputs=|+++
  plant : DiscreteStateSpace  A=Ad  B=Bd  C=eye(4)  D=zeros(4,2)  InitialCondition=x0_3  SampleTime=Ts
  sat_u : Saturate  UpperLimit=1.0  LowerLimit=-1.0
  sum2 : Sum  Inputs=|++
  sum3 : Sum  Inputs=|++
  ud_u1 : UnitDelay  InitialCondition=[0;0]  SampleTime=Ts  HasFrameUpgradeWarning=on
  ud_u2 : UnitDelay  InitialCondition=[0;0]  SampleTime=Ts  HasFrameUpgradeWarning=on
  ud_u3 : UnitDelay  InitialCondition=[0;0]  SampleTime=Ts  HasFrameUpgradeWarning=on
  ud_ua_prev : UnitDelay  InitialCondition=[0;0]  SampleTime=Ts  HasFrameUpgradeWarning=on
  uniformrandom : UniformRandomNumber  Minimum=0  SampleTime=Ts
  x_out : Outport
  ua_out : Outport  Port=2
  gamma_out : Outport  Port=3
  wires:
  ud_u1/1 -> ud_u2/1, DelaySel/2
  Relational Operator/1 -> gamma_out/1, Product_g/2, Gain_neg1/1
  ud_u3/1 -> DelaySel/4
  plant/1 -> Sum-e/1, x_out/1
  Produc_lt/1 -> sum3/2
  sum2/1 -> Produc_lt/1
  ud_ua_prev/1 -> Produc_lt/2
  Constant/1 -> sum2/2
  Gain_neg1/1 -> sum2/1
  DelaySel/1 -> Product_g/1
  Product_g/1 -> sum3/1
  ud_u2/1 -> ud_u3/1, DelaySel/3
  Sum-e/1 -> Gain_k/1
  sum3/1 -> ud_ua_prev/1, plant/1, ua_out/1
  uniformrandom/1 -> Relational Operator/1
  ref_in/1 -> Sum-e/2
  p_in/1 -> Relational Operator/2
  d_sel_in/1 -> DelaySel/1
  Gain_k/1 -> Sum_uc/1
  u_coop_in/1 -> Sum_uc/2
  Sum_uc/1 -> sat_u/1
  sat_u/1 -> ud_u1/1
  u_rep_in/1 -> Sum_uc/3

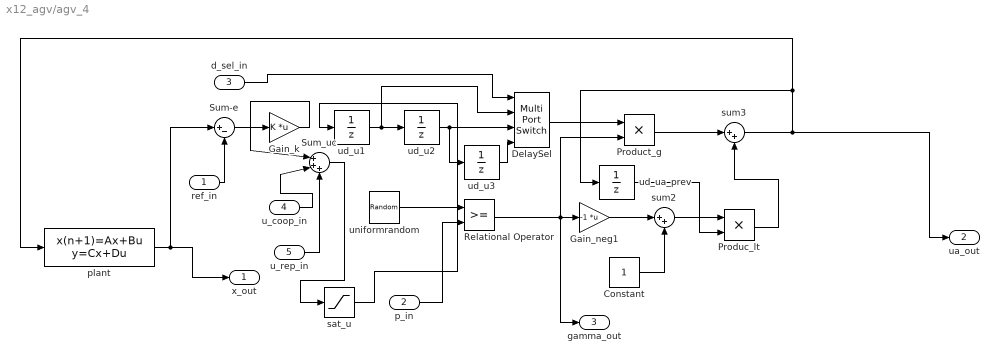
== system x12_agv/agv_4 ==
  ref_in : Inport
  p_in : Inport  Port=2
  d_sel_in : Inport  Port=3
  u_coop_in : Inport  Port=4
  u_rep_in : Inport  Port=5
  Constant : Constant
  DelaySel : MultiPortSwitch  DataPortOrder=Specify indices  DiagnosticForDefault=None  SaturateOnIntegerOverflow=off  InputSameDT=off
  Gain_k : Gain  Gain=K  Multiplication=Matrix(K*u)
  Gain_neg1 : Gain  Gain=-1  Multiplication=Matrix(K*u)
  Produc_lt : Product
  Product_g : Product
  Relational Operator : RelationalOperator  OutDataTypeStr=boolean  RndMeth=Simplest  InputSameDT=off
  Sum-e : Sum  Inputs=|+-
  Sum_uc : Sum  Inputs=|+++
  plant : DiscreteStateSpace  A=Ad  B=Bd  C=eye(4)  D=zeros(4,2)  InitialCondition=x0_4  SampleTime=Ts
  sat_u : Saturate  UpperLimit=1.0  LowerLimit=-1.0
  sum2 : Sum  Inputs=|++
  sum3 : Sum  Inputs=|++
  ud_u1 : UnitDelay  InitialCondition=[0;0]  SampleTime=Ts  HasFrameUpgradeWarning=on
  ud_u2 : UnitDelay  InitialCondition=[0;0]  SampleTime=Ts  HasFrameUpgradeWarning=on
  ud_u3 : UnitDelay  InitialCondition=[0;0]  SampleTime=Ts  HasFrameUpgradeWarning=on
  ud_ua_prev : UnitDelay  InitialCondition=[0;0]  SampleTime=Ts  HasFrameUpgradeWarning=on
  uniformrandom : UniformRandomNumber  Minimum=0  SampleTime=Ts
  x_out : Outport
  ua_out : Outport  Port=2
  gamma_out : Outport  Port=3
  wires:
  ud_u1/1 -> ud_u2/1, DelaySel/2
  Relational Operator/1 -> gamma_out/1, Product_g/2, Gain_neg1/1
  ud_u3/1 -> DelaySel/4
  plant/1 -> Sum-e/1, x_out/1
  Produc_lt/1 -> sum3/2
  sum2/1 -> Produc_lt/1
  ud_ua_prev/1 -> Produc_lt/2
  Constant/1 -> sum2/2
  Gain_neg1/1 -> sum2/1
  DelaySel/1 -> Product_g/1
  Product_g/1 -> sum3/1
  ud_u2/1 -> ud_u3/1, DelaySel/3
  Sum-e/1 -> Gain_k/1
  sum3/1 -> ud_ua_prev/1, plant/1, ua_out/1
  uniformrandom/1 -> Relational Operator/1
  ref_in/1 -> Sum-e/2
  p_in/1 -> Relational Operator/2
  d_sel_in/1 -> DelaySel/1
  Gain_k/1 -> Sum_uc/1
  u_coop_in/1 -> Sum_uc/2
  u_rep_in/1 -> Sum_uc/3
  Sum_uc/1 -> sat_u/1
  sat_u/1 -> ud_u1/1

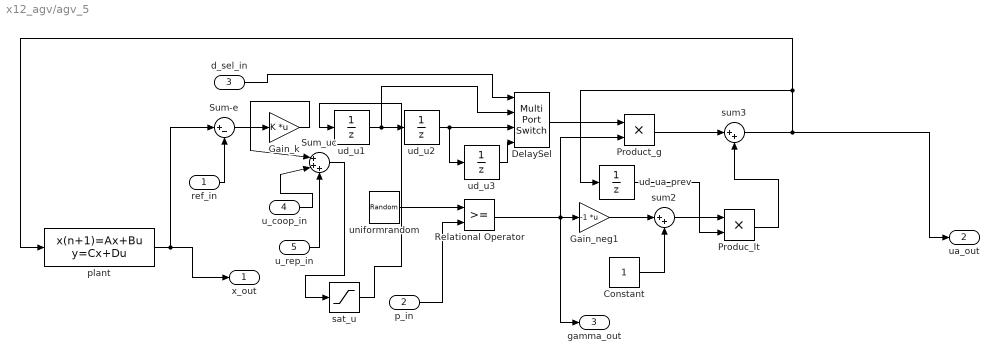
== system x12_agv/agv_5 ==
  ref_in : Inport
  p_in : Inport  Port=2
  d_sel_in : Inport  Port=3
  u_coop_in : Inport  Port=4
  u_rep_in : Inport  Port=5
  Constant : Constant
  DelaySel : MultiPortSwitch  DataPortOrder=Specify indices  DiagnosticForDefault=None  SaturateOnIntegerOverflow=off  InputSameDT=off
  Gain_k : Gain  Gain=K  Multiplication=Matrix(K*u)
  Gain_neg1 : Gain  Gain=-1  Multiplication=Matrix(K*u)
  Produc_lt : Product
  Product_g : Product
  Relational Operator : RelationalOperator  OutDataTypeStr=boolean  RndMeth=Simplest  InputSameDT=off
  Sum-e : Sum  Inputs=|+-
  Sum_uc : Sum  Inputs=|+++
  plant : DiscreteStateSpace  A=Ad  B=Bd  C=eye(4)  D=zeros(4,2)  InitialCondition=x0_5  SampleTime=Ts
  sat_u : Saturate  UpperLimit=1.0  LowerLimit=-1.0
  sum2 : Sum  Inputs=|++
  sum3 : Sum  Inputs=|++
  ud_u1 : UnitDelay  InitialCondition=[0;0]  SampleTime=Ts  HasFrameUpgradeWarning=on
  ud_u2 : UnitDelay  InitialCondition=[0;0]  SampleTime=Ts  HasFrameUpgradeWarning=on
  ud_u3 : UnitDelay  InitialCondition=[0;0]  SampleTime=Ts  HasFrameUpgradeWarning=on
  ud_ua_prev : UnitDelay  InitialCondition=[0;0]  SampleTime=Ts  HasFrameUpgradeWarning=on
  uniformrandom : UniformRandomNumber  Minimum=0  SampleTime=Ts
  x_out : Outport
  ua_out : Outport  Port=2
  gamma_out : Outport  Port=3
  wires:
  ud_u1/1 -> ud_u2/1, DelaySel/2
  Relational Operator/1 -> gamma_out/1, Product_g/2, Gain_neg1/1
  ud_u3/1 -> DelaySel/4
  plant/1 -> Sum-e/1, x_out/1
  Produc_lt/1 -> sum3/2
  sum2/1 -> Produc_lt/1
  ud_ua_prev/1 -> Produc_lt/2
  Constant/1 -> sum2/2
  Gain_neg1/1 -> sum2/1
  DelaySel/1 -> Product_g/1
  Product_g/1 -> sum3/1
  ud_u2/1 -> ud_u3/1, DelaySel/3
  Sum-e/1 -> Gain_k/1
  sum3/1 -> ud_ua_prev/1, plant/1, ua_out/1
  uniformrandom/1 -> Relational Operator/1
  ref_in/1 -> Sum-e/2
  p_in/1 -> Relational Operator/2
  d_sel_in/1 -> DelaySel/1
  Gain_k/1 -> Sum_uc/1
  u_coop_in/1 -> Sum_uc/2
  sat_u/1 -> ud_u1/1
  Sum_uc/1 -> sat_u/1
  u_rep_in/1 -> Sum_uc/3

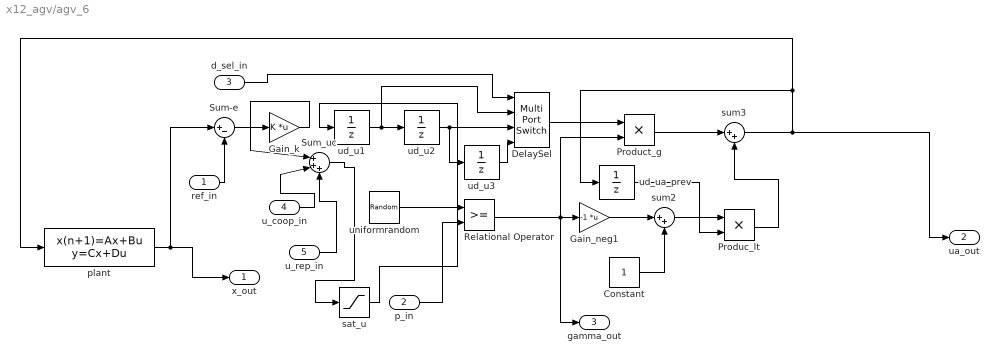
== system x12_agv/agv_6 ==
  ref_in : Inport
  p_in : Inport  Port=2
  d_sel_in : Inport  Port=3
  u_coop_in : Inport  Port=4
  u_rep_in : Inport  Port=5
  Constant : Constant
  DelaySel : MultiPortSwitch  DataPortOrder=Specify indices  DiagnosticForDefault=None  SaturateOnIntegerOverflow=off  InputSameDT=off
  Gain_k : Gain  Gain=K  Multiplication=Matrix(K*u)
  Gain_neg1 : Gain  Gain=-1  Multiplication=Matrix(K*u)
  Produc_lt : Product
  Product_g : Product
  Relational Operator : RelationalOperator  OutDataTypeStr=boolean  RndMeth=Simplest  InputSameDT=off
  Sum-e : Sum  Inputs=|+-
  Sum_uc : Sum  Inputs=|+++
  plant : DiscreteStateSpace  A=Ad  B=Bd  C=eye(4)  D=zeros(4,2)  InitialCondition=x0_6  SampleTime=Ts
  sat_u : Saturate  UpperLimit=1.0  LowerLimit=-1.0
  sum2 : Sum  Inputs=|++
  sum3 : Sum  Inputs=|++
  ud_u1 : UnitDelay  InitialCondition=[0;0]  SampleTime=Ts  HasFrameUpgradeWarning=on
  ud_u2 : UnitDelay  InitialCondition=[0;0]  SampleTime=Ts  HasFrameUpgradeWarning=on
  ud_u3 : UnitDelay  InitialCondition=[0;0]  SampleTime=Ts  HasFrameUpgradeWarning=on
  ud_ua_prev : UnitDelay  InitialCondition=[0;0]  SampleTime=Ts  HasFrameUpgradeWarning=on
  uniformrandom : UniformRandomNumber  Minimum=0  SampleTime=Ts
  x_out : Outport
  ua_out : Outport  Port=2
  gamma_out : Outport  Port=3
  wires:
  ud_u1/1 -> ud_u2/1, DelaySel/2
  Relational Operator/1 -> gamma_out/1, Product_g/2, Gain_neg1/1
  ud_u3/1 -> DelaySel/4
  plant/1 -> Sum-e/1, x_out/1
  Produc_lt/1 -> sum3/2
  sum2/1 -> Produc_lt/1
  ud_ua_prev/1 -> Produc_lt/2
  Constant/1 -> sum2/2
  Gain_neg1/1 -> sum2/1
  DelaySel/1 -> Product_g/1
  Product_g/1 -> sum3/1
  ud_u2/1 -> ud_u3/1, DelaySel/3
  Sum-e/1 -> Gain_k/1
  sum3/1 -> ud_ua_prev/1, plant/1, ua_out/1
  uniformrandom/1 -> Relational Operator/1
  ref_in/1 -> Sum-e/2
  p_in/1 -> Relational Operator/2
  d_sel_in/1 -> DelaySel/1
  Gain_k/1 -> Sum_uc/1
  u_coop_in/1 -> Sum_uc/2
  u_rep_in/1 -> Sum_uc/3
  Sum_uc/1 -> sat_u/1
  sat_u/1 -> ud_u1/1

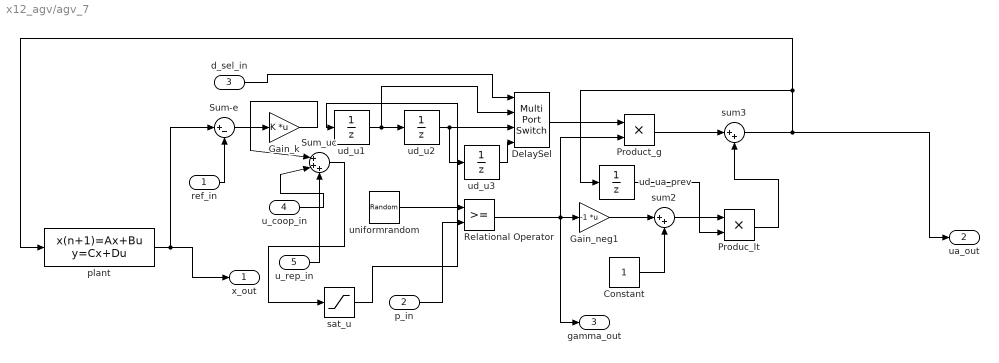
== system x12_agv/agv_7 ==
  ref_in : Inport
  p_in : Inport  Port=2
  d_sel_in : Inport  Port=3
  u_coop_in : Inport  Port=4
  u_rep_in : Inport  Port=5
  Constant : Constant
  DelaySel : MultiPortSwitch  DataPortOrder=Specify indices  DiagnosticForDefault=None  SaturateOnIntegerOverflow=off  InputSameDT=off
  Gain_k : Gain  Gain=K  Multiplication=Matrix(K*u)
  Gain_neg1 : Gain  Gain=-1  Multiplication=Matrix(K*u)
  Produc_lt : Product
  Product_g : Product
  Relational Operator : RelationalOperator  OutDataTypeStr=boolean  RndMeth=Simplest  InputSameDT=off
  Sum-e : Sum  Inputs=|+-
  Sum_uc : Sum  Inputs=|+++
  plant : DiscreteStateSpace  A=Ad  B=Bd  C=eye(4)  D=zeros(4,2)  InitialCondition=x0_7  SampleTime=Ts
  sat_u : Saturate  UpperLimit=1.0  LowerLimit=-1.0
  sum2 : Sum  Inputs=|++
  sum3 : Sum  Inputs=|++
  ud_u1 : UnitDelay  InitialCondition=[0;0]  SampleTime=Ts  HasFrameUpgradeWarning=on
  ud_u2 : UnitDelay  InitialCondition=[0;0]  SampleTime=Ts  HasFrameUpgradeWarning=on
  ud_u3 : UnitDelay  InitialCondition=[0;0]  SampleTime=Ts  HasFrameUpgradeWarning=on
  ud_ua_prev : UnitDelay  InitialCondition=[0;0]  SampleTime=Ts  HasFrameUpgradeWarning=on
  uniformrandom : UniformRandomNumber  Minimum=0  SampleTime=Ts
  x_out : Outport
  ua_out : Outport  Port=2
  gamma_out : Outport  Port=3
  wires:
  ud_u1/1 -> ud_u2/1, DelaySel/2
  Relational Operator/1 -> gamma_out/1, Product_g/2, Gain_neg1/1
  ud_u3/1 -> DelaySel/4
  plant/1 -> Sum-e/1, x_out/1
  Produc_lt/1 -> sum3/2
  sum2/1 -> Produc_lt/1
  ud_ua_prev/1 -> Produc_lt/2
  Constant/1 -> sum2/2
  Gain_neg1/1 -> sum2/1
  DelaySel/1 -> Product_g/1
  Product_g/1 -> sum3/1
  ud_u2/1 -> ud_u3/1, DelaySel/3
  Sum-e/1 -> Gain_k/1
  sum3/1 -> ud_ua_prev/1, plant/1, ua_out/1
  uniformrandom/1 -> Relational Operator/1
  ref_in/1 -> Sum-e/2
  p_in/1 -> Relational Operator/2
  d_sel_in/1 -> DelaySel/1
  Gain_k/1 -> Sum_uc/1
  u_coop_in/1 -> Sum_uc/2
  u_rep_in/1 -> Sum_uc/3
  Sum_uc/1 -> sat_u/1
  sat_u/1 -> ud_u1/1

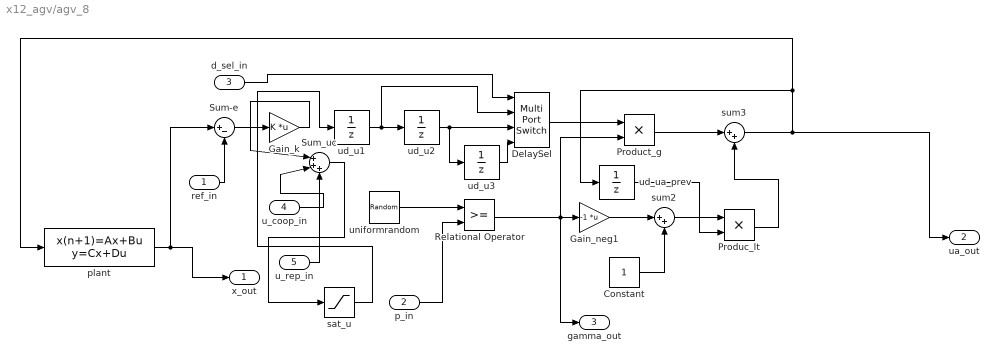
== system x12_agv/agv_8 ==
  ref_in : Inport
  p_in : Inport  Port=2
  d_sel_in : Inport  Port=3
  u_coop_in : Inport  Port=4
  u_rep_in : Inport  Port=5
  Constant : Constant
  DelaySel : MultiPortSwitch  DataPortOrder=Specify indices  DiagnosticForDefault=None  SaturateOnIntegerOverflow=off  InputSameDT=off
  Gain_k : Gain  Gain=K  Multiplication=Matrix(K*u)
  Gain_neg1 : Gain  Gain=-1  Multiplication=Matrix(K*u)
  Produc_lt : Product
  Product_g : Product
  Relational Operator : RelationalOperator  OutDataTypeStr=boolean  RndMeth=Simplest  InputSameDT=off
  Sum-e : Sum  Inputs=|+-
  Sum_uc : Sum  Inputs=|+++
  plant : DiscreteStateSpace  A=Ad  B=Bd  C=eye(4)  D=zeros(4,2)  InitialCondition=x0_8  SampleTime=Ts
  sat_u : Saturate  UpperLimit=1.0  LowerLimit=-1.0
  sum2 : Sum  Inputs=|++
  sum3 : Sum  Inputs=|++
  ud_u1 : UnitDelay  InitialCondition=[0;0]  SampleTime=Ts  HasFrameUpgradeWarning=on
  ud_u2 : UnitDelay  InitialCondition=[0;0]  SampleTime=Ts  HasFrameUpgradeWarning=on
  ud_u3 : UnitDelay  InitialCondition=[0;0]  SampleTime=Ts  HasFrameUpgradeWarning=on
  ud_ua_prev : UnitDelay  InitialCondition=[0;0]  SampleTime=Ts  HasFrameUpgradeWarning=on
  uniformrandom : UniformRandomNumber  Minimum=0  SampleTime=Ts
  x_out : Outport
  ua_out : Outport  Port=2
  gamma_out : Outport  Port=3
  wires:
  ud_u1/1 -> ud_u2/1, DelaySel/2
  Relational Operator/1 -> gamma_out/1, Product_g/2, Gain_neg1/1
  ud_u3/1 -> DelaySel/4
  plant/1 -> Sum-e/1, x_out/1
  Produc_lt/1 -> sum3/2
  sum2/1 -> Produc_lt/1
  ud_ua_prev/1 -> Produc_lt/2
  Constant/1 -> sum2/2
  Gain_neg1/1 -> sum2/1
  DelaySel/1 -> Product_g/1
  Product_g/1 -> sum3/1
  ud_u2/1 -> ud_u3/1, DelaySel/3
  Sum-e/1 -> Gain_k/1
  sum3/1 -> ud_ua_prev/1, plant/1, ua_out/1
  uniformrandom/1 -> Relational Operator/1
  ref_in/1 -> Sum-e/2
  p_in/1 -> Relational Operator/2
  d_sel_in/1 -> DelaySel/1
  Gain_k/1 -> Sum_uc/1
  u_coop_in/1 -> Sum_uc/2
  u_rep_in/1 -> Sum_uc/3
  sat_u/1 -> ud_u1/1
  Sum_uc/1 -> sat_u/1

== system x12_agv/agv_9 ==
  ref_in : Inport
  p_in : Inport  Port=2
  d_sel_in : Inport  Port=3
  u_coop_in : Inport  Port=4
  u_rep_in1 : Inport  Port=5
  Constant : Constant
  DelaySel : MultiPortSwitch  DataPortOrder=Specify indices  DiagnosticForDefault=None  SaturateOnIntegerOverflow=off  InputSameDT=off
  Gain_k : Gain  Gain=K  Multiplication=Matrix(K*u)
  Gain_neg1 : Gain  Gain=-1  Multiplication=Matrix(K*u)
  Produc_lt : Product
  Product_g : Product
  Relational Operator : RelationalOperator  OutDataTypeStr=boolean  RndMeth=Simplest  InputSameDT=off
  Sum-e : Sum  Inputs=|+-
  Sum_uc : Sum  Inputs=|+++
  plant : DiscreteStateSpace  A=Ad  B=Bd  C=eye(4)  D=zeros(4,2)  InitialCondition=x0_9  SampleTime=Ts
  sat_u1 : Saturate  UpperLimit=1.0  LowerLimit=-1.0
  sum2 : Sum  Inputs=|++
  sum3 : Sum  Inputs=|++
  ud_u1 : UnitDelay  InitialCondition=[0;0]  SampleTime=Ts  HasFrameUpgradeWarning=on
  ud_u2 : UnitDelay  InitialCondition=[0;0]  SampleTime=Ts  HasFrameUpgradeWarning=on
  ud_u3 : UnitDelay  InitialCondition=[0;0]  SampleTime=Ts  HasFrameUpgradeWarning=on
  ud_ua_prev : UnitDelay  InitialCondition=[0;0]  SampleTime=Ts  HasFrameUpgradeWarning=on
  uniformrandom : UniformRandomNumber  Minimum=0  SampleTime=Ts
  x_out : Outport
  ua_out : Outport  Port=2
  gamma_out : Outport  Port=3
  wires:
  ud_u1/1 -> ud_u2/1, DelaySel/2
  Relational Operator/1 -> gamma_out/1, Product_g/2, Gain_neg1/1
  ud_u3/1 -> DelaySel/4
  plant/1 -> Sum-e/1, x_out/1
  Produc_lt/1 -> sum3/2
  sum2/1 -> Produc_lt/1
  ud_ua_prev/1 -> Produc_lt/2
  Constant/1 -> sum2/2
  Gain_neg1/1 -> sum2/1
  DelaySel/1 -> Product_g/1
  Product_g/1 -> sum3/1
  ud_u2/1 -> ud_u3/1, DelaySel/3
  Sum-e/1 -> Gain_k/1
  sum3/1 -> ud_ua_prev/1, plant/1, ua_out/1
  uniformrandom/1 -> Relational Operator/1
  ref_in/1 -> Sum-e/2
  p_in/1 -> Relational Operator/2
  d_sel_in/1 -> DelaySel/1
  Gain_k/1 -> Sum_uc/1
  u_coop_in/1 -> Sum_uc/2
  u_rep_in1/1 -> Sum_uc/3
  Sum_uc/1 -> sat_u1/1
  sat_u1/1 -> ud_u1/1
